simulink subsystem "WFController"  (R2025b)
settings: Solver=VariableStepAuto  StartTime=0.0  StopTime=10.0  RelTol=1e-3
model mask{Kpv=0, Kiv=0, Kpicd=0, Kiicd=0, Kpicq=0, Kiicq=0, mVAbase=0, frequency=0, zBase=0, iMax=0, L=0, Kv=0}
  mask prompts: Kpv "Voltage Controller Proportional  Gain"; Kiv "Voltage Controller Integral  Gain"; Kpicd "D axis Proportional Gain"; Kiicd "D axis Integral Gain"; Kpicq "Q axis Proportional Gain"; Kiicq "Q axis Integral Gain"; mVAbase "Rated Power (VA)"; frequency "Rated Frequency (Hz)"; zBase "Base Impedance (Ohms)"; iMax "Maximum Current (PU)"; L "AC Filter Inductance (H)"; Kv "Rated AC Voltage (V)"
undefined symbols (not defined in the file): DiscIntNeverNeededParam, Kdv, sampleTime, Ts
libraries: slpidlib x2, eeTransforms x2
settings Model: Creator=rajarshd  LastModifiedBy=rajarshd

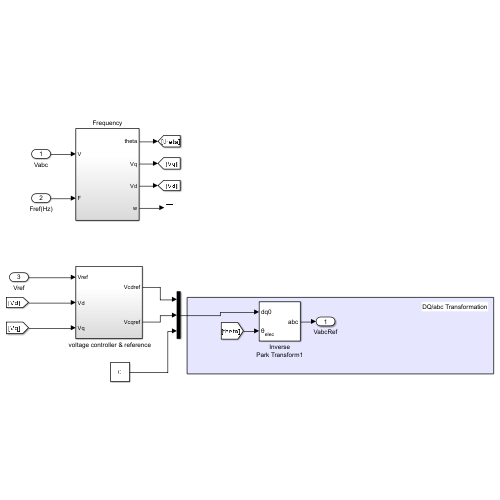
[thumbnail: Simulink's stored preview of the top-level diagram]
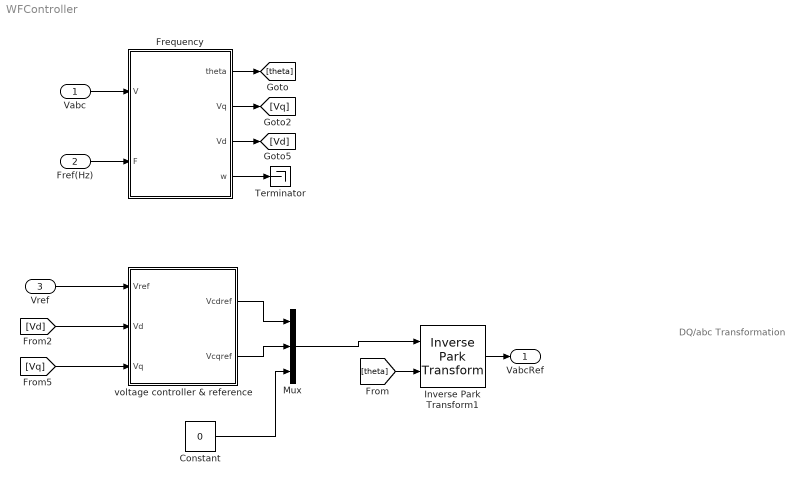
== system WFController ==
  note: DQ/abc Transformation
  Vabc : Inport
  Fref(Hz) : Inport  Port=2
  Vref : Inport  Port=3
  " voltage controller & reference" : Subsystem  SystemSampleTime=sampleTime
  Constant : Constant  Value=0
  Frequency : Subsystem
      settings: PortSchema="{\"entries\":[{\"content\":{\"sides\":[{\"content\":{\"connectorIds\":[\"Out1\",\"Out2\",\"Out3\",\"Out4\"]},\"type\":\"ConnectorPlacement.EquallySpacedRectSide\",\"uuid\":\"76485780-20fe-4fcf-8224-69648da6ed2a\"},{\"content\":{\"connectorIds\":[\"In1\",\"In2\"],\"side\":\"RIGHT\"},\"type\":\"ConnectorPlacement.EquallySpacedRectSide\",\"uuid\":\"f19a6390-e634-42c7-8d46-4cd80cbab182\"},{\"content\":{\"side\":\"TOP\"},\"type\":\"ConnectorPlacement.EquallySpacedRectSide\",\"uuid\":\"87682f72-1844-428e-be70-ad7ca3191ee3\"}]},\"type\":\"ConnectorPlacement.EquallySpacedConnector\",\"uuid\":\"f2136b07-48ec-402b-adb3-18c0bac2157c\"}],\"packageUris\":[\"http://schema.mathworks.com/mf0/Connector/R2020b\"],\"version\":\"1.0\"}"
  Inverse Park Transform1 : eeTransforms/Inverse Park Transform  AxisAlignment=Q-axis  PowerInvariant=off
  Mux : Mux  Inputs=3
  Terminator : Terminator
  VabcRef : Outport
  wires:
  Frequency/3(Vd) -> [Vd]
  Frequency/1(theta) -> [theta]
  Mux/1 -> Inverse Park Transform1/1
  [theta] -> Inverse Park Transform1/2
  Frequency/2(Vq) -> [Vq]
  Frequency/4(w) -> Terminator/1
  Vabc/1 -> Frequency/1(V)
  Fref(Hz)/1 -> Frequency/2(F)
  Vref/1 -> " voltage controller & reference"/1(Vref)
  [Vd] -> " voltage controller & reference"/2(Vd)
  [Vq] -> " voltage controller & reference"/3(Vq)
  " voltage controller & reference"/1(Vcdref) -> Mux/1
  " voltage controller & reference"/2(Vcqref) -> Mux/2
  Constant/1 -> Mux/3
  Inverse Park Transform1/1 -> VabcRef/1

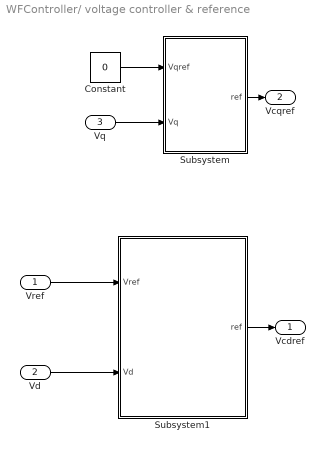
== system WFController/ voltage controller & reference ==
  Vref : Inport
  Vd : Inport  Port=2
  Vq : Inport  Port=3
  Constant : Constant  Value=0
  Subsystem : Subsystem
  Subsystem1 : Subsystem
  Vcdref : Outport
  Vcqref : Outport  Port=2
  wires:
  Subsystem1/1(ref) -> Vcdref/1
  Subsystem/1(ref) -> Vcqref/1
  Vq/1 -> Subsystem/2(Vq)
  Constant/1 -> Subsystem/1(Vqref)
  Vd/1 -> Subsystem1/2(Vd)
  Vref/1 -> Subsystem1/1(Vref)

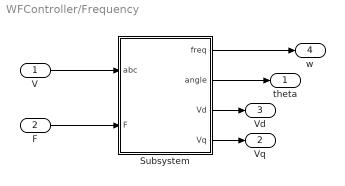
== system WFController/Frequency ==
  V : Inport
  F : Inport  Port=2
  Subsystem : Subsystem
  theta : Outport
  Vq : Outport  Port=2
  Vd : Outport  Port=3
  w : Outport  Port=4
  wires:
  F/1 -> Subsystem/2(F)
  V/1 -> Subsystem/1(abc)
  Subsystem/2(angle) -> theta/1
  Subsystem/4(Vq) -> Vq/1
  Subsystem/3(Vd) -> Vd/1
  Subsystem/1(freq) -> w/1

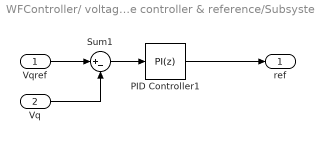
== system WFController/ voltage controller & reference/Subsystem ==
  Vqref : Inport
  Vq : Inport  Port=2
  PID Controller1 : slpidlib/PID Controller  Controller=PI  Form=Parallel  TimeDomain=Discrete-time  UseExternalTs=off  SampleTime=-1  IntegratorMethod=Forward Euler  FilterMethod=Forward Euler  ControllerParametersSource=internal  P=Kpv  I=Kiv  UseKiTs=off  D=Kdv  UseExternalDerivativeSource=off  N=100  UseFilter=on  TunerSelectOption=Transfer Function Based (PID Tuner App)  ZeroCross=off  InitialConditionSource=internal  InitialConditionForIntegrator=0  InitialConditionForFilter=0  DifferentiatorICPrevScaledInput=0  ExternalReset=none  TrackingMode=off  Kt=1  LimitOutput=off  SatLimitsSource=internal  UpperSaturationLimit=iMax  LowerSaturationLimit=0  LinearizeAsGain=on  AntiWindupMode=clamping  Kb=1  LimitIntegrator=off  UpperIntegratorSaturationLimit=inf  LowerIntegratorSaturationLimit=-inf  POutMin=[]  POutMax=[]  IOutMin=[]  IOutMax=[]  DOutMin=[]  DOutMax=[]  NOutMin=[]  NOutMax=[]  SumOutMin=[]  SumOutMax=[]  SaturationOutMin=[]  SaturationOutMax=[]  PParamMin=[]  PParamMax=[]  IParamMin=[]  IParamMax=[]  DParamMin=[]  DParamMax=[]  NParamMin=[]  NParamMax=[]  KbParamMin=[]  KbParamMax=[]  KtParamMin=[]  KtParamMax=[]  KbOutMin=[]  KbOutMax=[]  KtOutMin=[]  KtOutMax=[]  IntegratorOutMin=[]  IntegratorOutMax=[]  FilterOutMin=[]  FilterOutMax=[]  SumI1OutMin=[]  SumI1OutMax=[]  SumI2OutMin=[]  SumI2OutMax=[]  SumI3OutMin=[]  SumI3OutMax=[]  SumI4OutMin=[]  SumI4OutMax=[]  SumDOutMin=[]  SumDOutMax=[]  DifferentiatorOutMin=[]  DifferentiatorOutMax=[]  FilterDiffOutCoefMin=[]  FilterDiffOutCoefMax=[]  ReciprocalOutMin=[]  ReciprocalOutMax=[]  SumDenOutMin=[]  SumDenOutMax=[]  SumNumOutMin=[]  SumNumOutMax=[]  DivideOutMin=[]  DivideOutMax=[]  UdiffTsProdOutMin=[]  UdiffTsProdOutMax=[]  NTsProdOutMin=[]  NTsProdOutMax=[]  UintegralTsProdOutMin=[]  UintegralTsProdOutMax=[]  UngainTsProdOutMin=[]  UngainTsProdOutMax=[]  ClampingZeroOutDataTypeStr=Inherit: Inherit via back propagation  ClampingZeroOutMin=[]  ClampingZeroOutMax=[]  FilterDenConstantOutDataTypeStr=Inherit: Inherit via back propagation  FilterDenConstantOutMin=[]  FilterDenConstantOutMax=[]  PCopyOutDataTypeStr=Inherit: Inherit via back propagation  PCopyOutMin=[]  PCopyOutMax=[]  NCopyOutDataTypeStr=Inherit: Inherit via back propagation  NCopyOutMin=[]  NCopyOutMax=[]  IntegratorContinuousStateAttributes=''  IntegratorStateMustResolveToSignalObject=off  IntegratorRTWStateStorageClass=Auto  FilterContinuousStateAttributes=''  FilterStateMustResolveToSignalObject=off  FilterRTWStateStorageClass=Auto  ParallelPVariant=InternalParameters  IdealPVariant=Disabled  IVariant=InternalParameters  DVariant=Disabled  IntegratorVariant=Discrete  SatVariant=Disabled  AWVariant=Passthrough  PCopyVariant=Disabled  TRVariant=Disabled  FdbkBlocksVariant=Forward  IdealPFdbkVariant=Disabled  SatFdbkVariant=Disabled  DerivativeFilterVariant=Disabled  NVariant=Disabled  NCopyVariant=Disabled_SignalSpec  FilterICVariant=Disabled  IntegratorICVariant=InternalICs  ExternalResetVariant=Disabled  TRSumVariant=Passthrough  SumFdbkVariant=Disabled  SumVariant=Sum_PI  TsampFilterVariant=InternalTs  TsampNgainVariant=Passthrough  TsampIntegralVariant=Disabled_SignalSpec  ExternalSaturationOutDataTypeStr=Inherit: Same as second input  DerivativeSourceVariant=Disabled  PreIntVariant=InternalPreInt
  Sum1 : Sum  Inputs=|+-
  ref : Outport
  wires:
  PID Controller1/1 -> ref/1
  Vq/1 -> Sum1/2
  Vqref/1 -> Sum1/1
  Sum1/1 -> PID Controller1/1

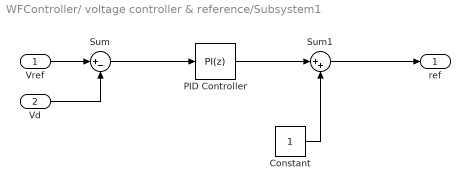
== system WFController/ voltage controller & reference/Subsystem1 ==
  Vref : Inport
  Vd : Inport  Port=2
  Constant : Constant
  PID Controller : slpidlib/PID Controller  Controller=PI  Form=Parallel  TimeDomain=Discrete-time  UseExternalTs=off  SampleTime=-1  IntegratorMethod=Forward Euler  FilterMethod=Forward Euler  ControllerParametersSource=internal  P=Kpv  I=Kiv  UseKiTs=off  D=Kdv  UseExternalDerivativeSource=off  N=100  UseFilter=on  TunerSelectOption=Transfer Function Based (PID Tuner App)  ZeroCross=off  InitialConditionSource=internal  InitialConditionForIntegrator=0  InitialConditionForFilter=0  DifferentiatorICPrevScaledInput=0  ExternalReset=none  TrackingMode=off  Kt=1  LimitOutput=off  SatLimitsSource=internal  UpperSaturationLimit=iMax  LowerSaturationLimit=0  LinearizeAsGain=on  AntiWindupMode=clamping  Kb=1  LimitIntegrator=off  UpperIntegratorSaturationLimit=inf  LowerIntegratorSaturationLimit=-inf  POutMin=[]  POutMax=[]  IOutMin=[]  IOutMax=[]  DOutMin=[]  DOutMax=[]  NOutMin=[]  NOutMax=[]  SumOutMin=[]  SumOutMax=[]  SaturationOutMin=[]  SaturationOutMax=[]  PParamMin=[]  PParamMax=[]  IParamMin=[]  IParamMax=[]  DParamMin=[]  DParamMax=[]  NParamMin=[]  NParamMax=[]  KbParamMin=[]  KbParamMax=[]  KtParamMin=[]  KtParamMax=[]  KbOutMin=[]  KbOutMax=[]  KtOutMin=[]  KtOutMax=[]  IntegratorOutMin=[]  IntegratorOutMax=[]  FilterOutMin=[]  FilterOutMax=[]  SumI1OutMin=[]  SumI1OutMax=[]  SumI2OutMin=[]  SumI2OutMax=[]  SumI3OutMin=[]  SumI3OutMax=[]  SumI4OutMin=[]  SumI4OutMax=[]  SumDOutMin=[]  SumDOutMax=[]  DifferentiatorOutMin=[]  DifferentiatorOutMax=[]  FilterDiffOutCoefMin=[]  FilterDiffOutCoefMax=[]  ReciprocalOutMin=[]  ReciprocalOutMax=[]  SumDenOutMin=[]  SumDenOutMax=[]  SumNumOutMin=[]  SumNumOutMax=[]  DivideOutMin=[]  DivideOutMax=[]  UdiffTsProdOutMin=[]  UdiffTsProdOutMax=[]  NTsProdOutMin=[]  NTsProdOutMax=[]  UintegralTsProdOutMin=[]  UintegralTsProdOutMax=[]  UngainTsProdOutMin=[]  UngainTsProdOutMax=[]  ClampingZeroOutDataTypeStr=Inherit: Inherit via back propagation  ClampingZeroOutMin=[]  ClampingZeroOutMax=[]  FilterDenConstantOutDataTypeStr=Inherit: Inherit via back propagation  FilterDenConstantOutMin=[]  FilterDenConstantOutMax=[]  PCopyOutDataTypeStr=Inherit: Inherit via back propagation  PCopyOutMin=[]  PCopyOutMax=[]  NCopyOutDataTypeStr=Inherit: Inherit via back propagation  NCopyOutMin=[]  NCopyOutMax=[]  IntegratorContinuousStateAttributes=''  IntegratorStateMustResolveToSignalObject=off  IntegratorRTWStateStorageClass=Auto  FilterContinuousStateAttributes=''  FilterStateMustResolveToSignalObject=off  FilterRTWStateStorageClass=Auto  ParallelPVariant=InternalParameters  IdealPVariant=Disabled  IVariant=InternalParameters  DVariant=Disabled  IntegratorVariant=Discrete  SatVariant=Disabled  AWVariant=Passthrough  PCopyVariant=Disabled  TRVariant=Disabled  FdbkBlocksVariant=Forward  IdealPFdbkVariant=Disabled  SatFdbkVariant=Disabled  DerivativeFilterVariant=Disabled  NVariant=Disabled  NCopyVariant=Disabled_SignalSpec  FilterICVariant=Disabled  IntegratorICVariant=InternalICs  ExternalResetVariant=Disabled  TRSumVariant=Passthrough  SumFdbkVariant=Disabled  SumVariant=Sum_PI  TsampFilterVariant=InternalTs  TsampNgainVariant=Passthrough  TsampIntegralVariant=Disabled_SignalSpec  ExternalSaturationOutDataTypeStr=Inherit: Same as second input  DerivativeSourceVariant=Disabled  PreIntVariant=InternalPreInt
  Sum : Sum  Inputs=|+-
  Sum1 : Sum  Inputs=|++
  ref : Outport
  wires:
  PID Controller/1 -> Sum1/1
  Sum1/1 -> ref/1
  Constant/1 -> Sum1/2
  Vd/1 -> Sum/2
  Vref/1 -> Sum/1
  Sum/1 -> PID Controller/1

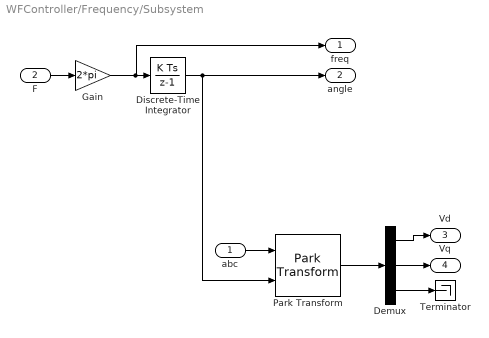
== system WFController/Frequency/Subsystem ==
  abc : Inport
  F : Inport  Port=2
  Demux : Demux  Outputs=3
  Discrete-Time Integrator : DiscreteIntegrator  SampleTime=Ts  ICPrevOutput=DiscIntNeverNeededParam  ICPrevScaledInput=DiscIntNeverNeededParam
  Gain : Gain  Gain=2*pi
  Park Transform : eeTransforms/Park Transform  AxisAlignment=Q-axis  PowerInvariant=off
  Terminator : Terminator
  freq : Outport
  angle : Outport  Port=2
  Vd : Outport  Port=3
  Vq : Outport  Port=4
  wires:
  Gain/1 -> Discrete-Time Integrator/1, freq/1
  Demux/3 -> Terminator/1
  abc/1 -> Park Transform/1
  Park Transform/1 -> Demux/1
  Demux/1 -> Vd/1
  Demux/2 -> Vq/1
  F/1 -> Gain/1
  Discrete-Time Integrator/1 -> Park Transform/2, angle/1
